simulink model "PowerSystem_FinalProject"  (R2020b)
settings: Solver=ode8  StartTime=0.0  StopTime=10  RelTol=1e-4  EnableMultiTasking=on
PreLoadFcn:
  | ct = 1.083
undefined symbols (not defined in the file): D1, Delta
libraries: powerlib x43, powerlib_meascontrol x9, sps_avr x3
settings Model: Creator=jp536285  LastModifiedBy=Arda
settings DataIOCC: SaveFormat=Array  SaveOutput=off  SaveTime=off  ReturnWorkspaceOutputs=off
settings OptimizationCC: LifeSpan=inf
settings DebuggingCC: UnderspecifiedInitializationDetection=Classic  MergeDetectMultiDrivingBlocksExec=none  SolverPrmCheckMsg=warning  UnconnectedInputMsg=none  UnconnectedOutputMsg=none  UnconnectedLineMsg=none  StateNameClashWarn=warning  SFUnexpectedBacktrackingDiag=warning  SFNoUnconditionalDefaultTransitionDiag=warning  SFExecutionAtInitializationDiag=none  ArithmeticOperatorsInVariantConditions=warning
settings HardwareCC: ProdBitPerPointer=32  ProdBitPerSizeT=32  ProdBitPerPtrDiffT=32  ProdLargestAtomicFloat=None  ProdIntDivRoundTo=Undefined  ProdEndianess=Unspecified  ProdWordSize=32  ProdHWDeviceType=32-bit Generic
settings ModelReferenceCC: PropagateSignalLabelsOutOfModel=off
settings SFSimCC: SimUseLocalCustomCode=off  CustomCodeUndefinedFunction=UseInterfaceOnly
settings RTWCC: RTWUseLocalCustomCode=off
settings CodeAppCC: StateflowObjectComments=on
settings GRTTargetCC: TargetLangStandard=C89/C90 (ANSI)
settings ConfigComp: CovMetricSettings=dw  CovSaveCumulativeToWorkspaceVar=on  CovSaveSingleToWorkspaceVar=on  CovExternalEMLEnable=off
settings SimscapeCC: SimscapeNormalizeSystem=off

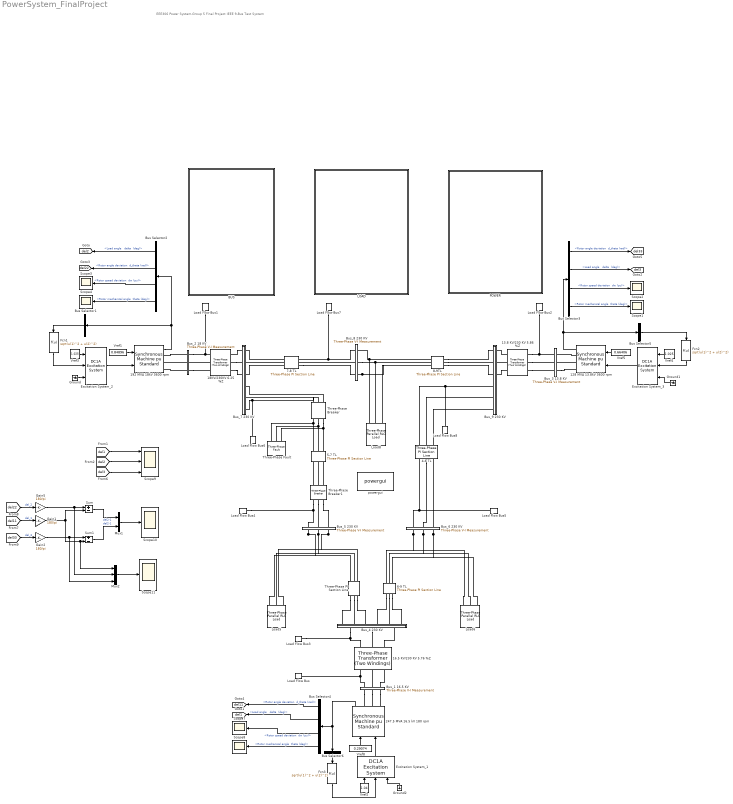
== system PowerSystem_FinalProject ==
  note: EEE306 Power System-Group 5
      |                      Final Project
      |             IEEE 9-Bus Test System
  128 MVA 13.8kV 3600 rpm : powerlib/Machines/Synchronous Machine pu Standard  PresetModel=No  MechanicalLoad=Mechanical power Pm  ShowDetailedParameters=on  RotorType=Round  Units=per unit standard parameters  MeasurementBus=off  NominalParameters="[ 128e6  13.8e3   60 ]"  Reactances1=[ 1.68, 0.23206, 0.19, 1.61, 0.23206, 0.19, 0.314]  Reactances2="[ 1.305, 0.296, 0.252, 0.474,  0.243,  0.18 ]"  dAxisTimeConstants=Open-circuit  qAxisTimeConstants=Open-circuit  TimeConstants1="[ 4.4849  0.0681  0.1  ]"  TimeConstants2=[ 5.89, 0.001,0.6, 0.001 ]  TimeConstants3="[  4.49  0.0681  0.0513  ]"  TimeConstants4=[ 8.0, 0.03, 0.3371, 0.0295 ]  TimeConstants5=[ 1.01, 0.053, 0.1 ]  TimeConstants6=[ 1.3201, 0.023, 1.0, 0.07 ]  TimeConstants7="[  1.01  0.053  0.051266  ]"  TimeConstants8=[ 1.3201, 0.0231, 0.3371, 0.0295 ]  StatorResistance=1e-7  Mechanical="[ 2.35  0 1 ]"  PolePairs=1  InitialConditions=[0 -40.1892 0.648353 0.648353 0.648353 5.37848 -114.622 125.378 1.46611]  SetSaturation=off  Saturation=[0.6404,0.7127,0.8441,0.9214,0.9956,1.082,1.19,1.316,1.457;0.7,0.7698,0.8872,0.9466,0.9969,1.046,1.1,1.151,1.201]  LoadFlowParameters=[1 85000000 0 0 0]  TsPowergui=0  TsBlock=-1  IterativeModel=Trapezoidal non iterative  IterativeDiscreteModel=Trapezoidal non iterative  BusType=PV  Pref=85000000  Qref=0  Qmin=-Inf  Qmax=Inf  PLF=0  QLF=0
  13.8 KV/230 KV 5.86 %Z : powerlib/Elements/Three-Phase Transformer (Two Windings)  Winding1Connection=Delta (D1)  Winding2Connection=Yg  CoreType=Three single-phase transformers  SetSaturation=off  Hysteresis=off  DataFile='hysteresis'  SetInitialFlux=off  Measurements=None  UNITS=pu  NominalPower=[ 128e6 , 60 ]  Winding1=[ 13.8e3 , 1e-6 , 0 ]  Winding2=[ 230e3 , 1e-6, 0.0586 ]  Rm=500  Lm=500  L0=0.5  Saturation=[ 0,0 ; 0.0024,1.2 ; 1.0,1.52 ]  InitialFluxes=[ 0.8 , -0.8 , 0.7 ]  BreakLoop=off  DiscreteSolver=Trapezoidal iterative  DataType=off  TransfoNumber=1
  "16.5 KV/230 KV 5.76 %Z     " : powerlib/Elements/Three-Phase Transformer (Two Windings)  Winding1Connection=Delta (D1)  Winding2Connection=Yg  CoreType=Three single-phase transformers  SetSaturation=off  Hysteresis=off  DataFile='hysteresis'  SetInitialFlux=off  Measurements=None  UNITS=pu  NominalPower=[ 247.5e6 , 60 ]  Winding1=[ 16.5e3 , 1e-6, 0 ]  Winding2=[ 230e3 ,1e-6, 0.0576 ]  Rm=500  Lm=500  L0=0.5  Saturation=[ 0,0 ; 0.0024,1.2 ; 1.0,1.52 ]  InitialFluxes=[ 0.8 , -0.8 , 0.7 ]  BreakLoop=off  DiscreteSolver=Trapezoidal iterative  DataType=off  TransfoNumber=1
  18KV/230KV 6.25 %Z : powerlib/Elements/Three-Phase Transformer (Two Windings)  Winding1Connection=Delta (D1)  Winding2Connection=Yg  CoreType=Three single-phase transformers  SetSaturation=off  Hysteresis=off  DataFile='hysteresis'  SetInitialFlux=off  Measurements=None  UNITS=pu  NominalPower=[ 192e6, 60 ]  Winding1=[ 18e3 , 1e-6 , 0]  Winding2=[ 230e3 , 1e-6, 0.0625 ]  Rm=500  Lm=500  L0=0.5  Saturation=[ 0,0 ; 0.0024,1.2 ; 1.0,1.52 ]  InitialFluxes=[ 0.8 , -0.8 , 0.7 ]  BreakLoop=off  DiscreteSolver=Trapezoidal iterative  DataType=off  TransfoNumber=1
  192 MVA 18kV 3600 rpm : powerlib/Machines/Synchronous Machine pu Standard  PresetModel=No  MechanicalLoad=Mechanical power Pm  ShowDetailedParameters=on  RotorType=Round  Units=per unit standard parameters  MeasurementBus=off  NominalParameters="[ 192e6  18e3   60 ]"  Reactances1=[ 1.72, 0.23, 0.1728,1.65, 0.23, 0.1728, 0.4224 ]  Reactances2="[ 1.305, 0.296, 0.252, 0.474,  0.243,  0.18 ]"  dAxisTimeConstants=Open-circuit  qAxisTimeConstants=Open-circuit  TimeConstants1="[ 4.4849  0.0681  0.1  ]"  TimeConstants2=[ 6, 0.001, 0.53, 0.001]  TimeConstants3="[  4.49  0.0681  0.0513  ]"  TimeConstants4=[ 8.0, 0.03, 0.3371, 0.0295 ]  TimeConstants5=[ 1.01, 0.053, 0.1 ]  TimeConstants6=[ 1.3201, 0.023, 1.0, 0.07 ]  TimeConstants7="[  1.01  0.053  0.051266  ]"  TimeConstants8=[ 1.3201, 0.0231, 0.3371, 0.0295 ]  StatorResistance=1e-7  Mechanical="[ 3.33  0 1 ]"  PolePairs=1  InitialConditions=[0 -30.0005 0.828257 0.828257 0.828257 6.94163 -113.058 126.942 1.7518]  SetSaturation=off  Saturation=[0.6404,0.7127,0.8441,0.9214,0.9956,1.082,1.19,1.316,1.457;0.7,0.7698,0.8872,0.9466,0.9969,1.046,1.1,1.151,1.201]  LoadFlowParameters=[1 163000000 0 0 0]  TsPowergui=0  TsBlock=-1  IterativeModel=Trapezoidal non iterative  IterativeDiscreteModel=Trapezoidal non iterative  BusType=PV  Pref=163000000  Qref=0  Qmin=-Inf  Qmax=Inf  PLF=0  QLF=0
  247.5 MVA 16.5 kV 180 rpm : powerlib/Machines/Synchronous Machine pu Standard  PresetModel=No  MechanicalLoad=Mechanical power Pm  ShowDetailedParameters=on  RotorType=Salient-pole  Units=per unit standard parameters  MeasurementBus=off  NominalParameters="[ 247.5e6  16500   60 ]"  Reactances1=[ 31 32 33 34 35 36 37 ]  Reactances2=[ 0.361, 0.1504, 0.099, 0.2398, 0.099, 0.062 ]  dAxisTimeConstants=Open-circuit  qAxisTimeConstants=Open-circuit  TimeConstants1=[8.96 0.001 0.001]  TimeConstants2=[]  TimeConstants3=[]  TimeConstants4=[]  TimeConstants5=[ 1.01, 0.053, 0.31 ]  TimeConstants6=[]  TimeConstants7=[]  TimeConstants8=[]  StatorResistance=1e-7  Mechanical=[9.55 0 20]  PolePairs=20  InitialConditions=[0 -86.3582 0.284957 0.284957 0.284957 -11.1761 -131.176 108.824 1.06421]  SetSaturation=off  Saturation=[0.6404,0.7127,0.8441,0.9214,0.9956,1.082,1.19,1.316,1.457;0.7,0.7698,0.8872,0.9466,0.9969,1.046,1.1,1.151,1.201]  LoadFlowParameters=[2 71000000 0 0]  TsPowergui=0  TsBlock=-1  IterativeModel=Trapezoidal non iterative  IterativeDiscreteModel=Trapezoidal non iterative  BusType=swing  Pref=150000000  Qref=0  Qmin=-Inf  Qmax=Inf  PLF=0  QLF=0
      settings: AttributesFormatString=\n\n
  4-6 TL : powerlib/Elements/Three-Phase PI Section Line  LConnTagsString=a|b|c  RConnTagsString=A|B|C  Length=97.336  Frequency=60  Resistances=[9.24e-2 9.24e-1]  Inductances=[1.40e-3 3.98e-3]  Capacitances=[8.14e-9 4.88e-9]
  5-7 TL : powerlib/Elements/Three-Phase PI Section Line  LConnTagsString=a|b|c  RConnTagsString=A|B|C  Length=170.338  Frequency=60  Resistances=[9.94e-2 9.94e-1]  Inductances=[1.4e-3 3.98e-3]  Capacitances=[9.01e-9 5.41e-9]
  6-9 TL : powerlib/Elements/Three-Phase PI Section Line  LConnTagsString=a|b|c  RConnTagsString=A|B|C  Length=179.86  Frequency=60  Resistances=[1.15e-1 1.15]  Inductances=[1.4e-3 3.98e-3]  Capacitances=[9.98e-9 5.99e-9]
  7-8 TL : powerlib/Elements/Three-Phase PI Section Line  LConnTagsString=a|b|c  RConnTagsString=A|B|C  Length=76.176  Frequency=60  Resistances=[5.90e-2 5.90e-1]  Inductances=[1.4e-3 3.98e-3]  Capacitances=[9.81e-9 5.89e-9]
  8-9TL : powerlib/Elements/Three-Phase PI Section Line  LConnTagsString=a|b|c  RConnTagsString=A|B|C  Length=106.646  Frequency=60  Resistances=[5.9e-2 5.9e-1]  Inductances=[1.4e-3 3.98e-3]  Capacitances=[9.83e-9 5.9e-9]
  "BUS " : Subsystem
  Bus Selector1 : BusSelector  OutputSignals="dq0 components.Stator voltage  vq (pu),dq0 components.Stator voltage  vd (pu)"  OutputAsBus=on
  Bus Selector2 : BusSelector  OutputSignals="Load angle   delta  (deg),Mechanical.Rotor angle deviation  d_theta (rad),Mechanical.Rotor speed deviation  dw (pu),Mechanical.Rotor mechanical angle  theta (deg)"
  Bus Selector3 : BusSelector  OutputSignals="Mechanical.Rotor angle deviation  d_theta (rad),Load angle   delta  (deg),Mechanical.Rotor speed deviation  dw (pu),Mechanical.Rotor mechanical angle  theta (deg)"
  Bus Selector4 : BusSelector  OutputSignals="Mechanical.Rotor angle deviation  d_theta (rad),Load angle   delta  (deg),Mechanical.Rotor speed deviation  dw (pu),Mechanical.Rotor mechanical angle  theta (deg)"
  Bus Selector5 : BusSelector  OutputSignals="dq0 components.Stator voltage  vq (pu),dq0 components.Stator voltage  vd (pu)"  OutputAsBus=on
  Bus Selector6 : BusSelector  OutputSignals="dq0 components.Stator voltage  vq (pu),dq0 components.Stator voltage  vd (pu)"  OutputAsBus=on
  Bus_1 16.5 KV : powerlib/Measurements/Three-Phase V-I Measurement  VoltageMeasurement=phase-to-phase  SetLabelV=on  LabelV=Vabc_1  Vpu=on  VpuLL=off  CurrentMeasurement=yes  SetLabelI=on  LabelI=Iabc_1  Ipu=on  Pbase=100e6  Vbase=16.5e3  OutputType=Complex  PhasorSimulation=off  PSBequivalent=0
  Bus_2 18 KV : powerlib/Measurements/Three-Phase V-I Measurement  VoltageMeasurement=phase-to-phase  SetLabelV=on  LabelV=Vabc_2  Vpu=on  VpuLL=off  CurrentMeasurement=yes  SetLabelI=on  LabelI=Iabc_2  Ipu=on  Pbase=100e6  Vbase=18e3  OutputType=Complex  PhasorSimulation=off  PSBequivalent=0
  Bus_3 13.8 KV : powerlib/Measurements/Three-Phase V-I Measurement  VoltageMeasurement=phase-to-phase  SetLabelV=on  LabelV=Vabc_3  Vpu=on  VpuLL=off  CurrentMeasurement=yes  SetLabelI=on  LabelI=Iabc_3  Ipu=on  Pbase=100e6  Vbase=13.8e3  OutputType=Complex  PhasorSimulation=off  PSBequivalent=0
  Bus_4 230 KV : Subsystem
  Bus_5 230 KV : powerlib/Measurements/Three-Phase V-I Measurement  VoltageMeasurement=phase-to-ground  SetLabelV=on  LabelV=Vabc_5  Vpu=on  VpuLL=off  CurrentMeasurement=yes  SetLabelI=on  LabelI=Iabc_5  Ipu=on  Pbase=100e6  Vbase=230e3  OutputType=Complex  PhasorSimulation=off  PSBequivalent=0
  Bus_6 230 KV : powerlib/Measurements/Three-Phase V-I Measurement  VoltageMeasurement=phase-to-ground  SetLabelV=on  LabelV=Vabc_6  Vpu=on  VpuLL=off  CurrentMeasurement=yes  SetLabelI=on  LabelI=Iabc_6  Ipu=on  Pbase=100e6  Vbase=230e3  OutputType=Complex  PhasorSimulation=off  PSBequivalent=0
  Bus_7 230 KV : Subsystem
  Bus_8 230 KV : powerlib/Measurements/Three-Phase V-I Measurement  VoltageMeasurement=phase-to-ground  SetLabelV=on  LabelV=Vabc_8  Vpu=on  VpuLL=off  CurrentMeasurement=yes  SetLabelI=on  LabelI=Iabc_8  Ipu=on  Pbase=100e6  Vbase=230e3  OutputType=Complex  PhasorSimulation=off  PSBequivalent=0
  Bus_9 230 KV : Subsystem
  Excitation System_2 : sps_avr/DC1A Excitation System  Tr=20e-3  KaTa=[20 0.2]  VRminmax=[ -4 4]  KfTf=[0.063 0.35]  TbTc=[0 0]  KeTe=[1 0.314]  Efd12=[3.1 2.3]  SeEfd12=[0.483 0.1394]  v0=[1.025 1.7518]  TsBlock=0
      settings: SourceProductBaseCode=PS
  Excitation System_1 : sps_avr/DC1A Excitation System  Tr=20e-3  KaTa=[20 0.2]  VRminmax=[ -3 3]  KfTf=[0.063 0.35]  TbTc=[0 0]  KeTe=[1 0.314]  Efd12=[3.1 2.3]  SeEfd12=[0.483 0.1394]  v0=[1.04 1.0642]  TsBlock=0
      settings: SourceProductBaseCode=PS
  Excitation System_3 : sps_avr/DC1A Excitation System  Tr=20e-3  KaTa=[20 0.2]  VRminmax=[-4 4]  KfTf=[0.063 0.35]  TbTc=[0 0]  KeTe=[1 0.314]  Efd12=[3.1 2.3]  SeEfd12=[0.483 0.1394]  v0=[1.025 1.4661]  TsBlock=0
      settings: SourceProductBaseCode=PS
  Fcn1 : Fcn  Expr=sqrt(u(1)^2 + u(2)^2)
  Fcn2 : Fcn  Expr=sqrt(u(1)^2 + u(2)^2)
  Fcn3 : Fcn  Expr=sqrt(u(1)^2 + u(2)^2)
  Gain1 : Gain  Gain=180/pi
  Gain2 : Gain  Gain=180/pi
  Gain5 : Gain  Gain=180/pi
  Ground : Ground
  Ground1 : Ground
  Ground2 : Ground
  LOAD : Subsystem
  Load Flow Bus : powerlib/Measurements/Load Flow Bus  LConnTagsString=a  Phases=single  Connectors=on one side  ID=BUS_1  Vbase=16.5e3  Vref=1.04  Vangle=0  VLF=1.04  VLFb=1  VLFc=1  angleLF=0  angleLFb=0  angleLFc=0
      settings: AttributesFormatString=%<ID>\n%<Vbase>V\n%<VLF>pu\n%<angleLF>deg.
  Load Flow Bus1 : powerlib/Measurements/Load Flow Bus  LConnTagsString=a  Phases=single  Connectors=on one side  ID=BUS_2  Vbase=18e3  Vref=1.025  Vangle=0  VLF=1.025  VLFb=1  VLFc=1  angleLF=6.743  angleLFb=0  angleLFc=0
      settings: AttributesFormatString=%<ID>\n%<Vbase>V\n%<VLF>pu\n%<angleLF>deg.
  Load Flow Bus2 : powerlib/Measurements/Load Flow Bus  LConnTagsString=a  Phases=single  Connectors=on one side  ID=BUS_3  Vbase=13.8e3  Vref=1.025  Vangle=0  VLF=1.025  VLFb=1  VLFc=1  angleLF=3.158  angleLFb=0  angleLFc=0
      settings: AttributesFormatString=%<ID>\n%<Vbase>V\n%<VLF>pu\n%<angleLF>deg.
  Load Flow Bus3 : powerlib/Measurements/Load Flow Bus  LConnTagsString=a  Phases=single  Connectors=on one side  ID=BUS_4  Vbase=230e3  Vref=1  Vangle=0  VLF=1.037  VLFb=1  VLFc=1  angleLF=29.12  angleLFb=0  angleLFc=0
      settings: AttributesFormatString=%<ID>\n%<Vbase>V\n%<VLF>pu\n%<angleLF>deg.
  Load Flow Bus4 : powerlib/Measurements/Load Flow Bus  LConnTagsString=a  Phases=single  Connectors=on one side  ID=BUS_5  Vbase=230e3  Vref=1  Vangle=0  VLF=1.004  VLFb=1  VLFc=1  angleLF=26.79  angleLFb=0  angleLFc=0
      settings: AttributesFormatString=%<ID>\n%<Vbase>V\n%<VLF>pu\n%<angleLF>deg.
  Load Flow Bus5 : powerlib/Measurements/Load Flow Bus  LConnTagsString=a  Phases=single  Connectors=on one side  ID=BUS_6  Vbase=230e3  Vref=1  Vangle=0  VLF=1.017  VLFb=1  VLFc=1  angleLF=27.3  angleLFb=0  angleLFc=0
      settings: AttributesFormatString=%<ID>\n%<Vbase>V\n%<VLF>pu\n%<angleLF>deg.
  Load Flow Bus6 : powerlib/Measurements/Load Flow Bus  LConnTagsString=a  Phases=single  Connectors=on one side  ID=BUS_7  Vbase=230e3  Vref=1  Vangle=0  VLF=1.027  VLFb=1  VLFc=1  angleLF=33.86  angleLFb=0  angleLFc=0
      settings: AttributesFormatString=%<ID>\n%<Vbase>V\n%<VLF>pu\n%<angleLF>deg.
  Load Flow Bus7 : powerlib/Measurements/Load Flow Bus  LConnTagsString=a  Phases=single  Connectors=on one side  ID=BUS_8  Vbase=230e3  Vref=1  Vangle=0  VLF=1.014  VLFb=1  VLFc=1  angleLF=30.3  angleLFb=0  angleLFc=0
      settings: AttributesFormatString=%<ID>\n%<Vbase>V\n%<VLF>pu\n%<angleLF>deg.
  Load Flow Bus8 : powerlib/Measurements/Load Flow Bus  LConnTagsString=a  Phases=single  Connectors=on one side  ID=BUS_9  Vbase=230e3  Vref=1  Vangle=0  VLF=1.027  VLFb=1  VLFc=1  angleLF=31.05  angleLFb=0  angleLFc=0
      settings: AttributesFormatString=%<ID>\n%<Vbase>V\n%<VLF>pu\n%<angleLF>deg.
  Load5 : powerlib/Elements/Three-Phase Parallel RLC Load  LConnTagsString=A|B|C  Configuration=Y (grounded)  NominalVoltage=(230000)*1.00389  Vabc=[1e3 1e3 1e3]  Vabcp=[1e3 1e3 1e3]  NominalFrequency=60  UnbalancedPower=off  ActivePower=125e6  InductivePower=50e6  CapacitivePower=0  Pabc=[10e3 9e3 11e3]  QLabc=[100 90 110]  QCabc=[100 90 110]  Pabcp=[10e3 9e3 11e3]  QLabcp=[100 90 110]  QCabcp=[100 90 110]  Measurements=Branch voltages and currents  LoadType=constant PQ
  Load6 : powerlib/Elements/Three-Phase Parallel RLC Load  LConnTagsString=A|B|C  Configuration=Y (grounded)  NominalVoltage=(230000)*1.01696  Vabc=[1e3 1e3 1e3]  Vabcp=[1e3 1e3 1e3]  NominalFrequency=60  UnbalancedPower=off  ActivePower=90e6  InductivePower=30e6  CapacitivePower=0  Pabc=[10e3 9e3 11e3]  QLabc=[100 90 110]  QCabc=[100 90 110]  Pabcp=[10e3 9e3 11e3]  QLabcp=[100 90 110]  QCabcp=[100 90 110]  Measurements=Branch voltages and currents  LoadType=constant PQ
  Load8 : powerlib/Elements/Three-Phase Parallel RLC Load  LConnTagsString=A|B|C  Configuration=Y (grounded)  NominalVoltage=(230000)*1.0136  Vabc=[1e3 1e3 1e3]  Vabcp=[1e3 1e3 1e3]  NominalFrequency=60  UnbalancedPower=off  ActivePower=100e6  InductivePower=35e6  CapacitivePower=0  Pabc=[10e3 9e3 11e3]  QLabc=[100 90 110]  QCabc=[100 90 110]  Pabcp=[10e3 9e3 11e3]  QLabcp=[100 90 110]  QCabcp=[100 90 110]  Measurements=Branch voltages and currents  LoadType=constant PQ
  Mux1 : Mux  Inputs=2
  Mux2 : Mux  Inputs=3
  POWER : Subsystem
  Scope{1..4,7..8,10..11} (8 alike) : Scope
  Scope9 : Scope  NumInputPorts=3
  Sum : Sum  Inputs=+-
  Sum1 : Sum  Inputs=+-
  Three-Phase PI Section Line : powerlib/Elements/Three-Phase PI Section Line  LConnTagsString=a|b|c  RConnTagsString=A|B|C  Length=89.93  Frequency=60  Resistances=[5.88e-2 5.88e-1]  Inductances=[1.4e-3 3.98e-3]  Capacitances=[9.81e-9 5.89e-9]
  Three-Phase Breaker : powerlib/Elements/Three-Phase Breaker  InitialState=closed  SwitchA=on  SwitchB=on  SwitchC=on  SwitchTimes=[ct]  External=off  BreakerResistance=0.001  SnubberResistance=1e7  SnubberCapacitance=inf  Measurements=None
  Three-Phase Breaker1 : powerlib/Elements/Three-Phase Breaker  InitialState=closed  SwitchA=on  SwitchB=on  SwitchC=on  SwitchTimes=[ct]  External=off  BreakerResistance=0.001  SnubberResistance=1e7  SnubberCapacitance=inf  Measurements=None
  Three-Phase Fault : powerlib/Elements/Three-Phase Fault  InitialStates=0  FaultA=on  FaultB=on  FaultC=on  GroundFault=on  SwitchTimes=[1 ct]  External=off  SwitchStatus=NaN  FaultResistance=0.001  GroundResistance=0.01  SnubberResistance=1e6  SnubberCapacitance=inf  Measurements=None
  Vref1 : Constant  Value=0.84896
  Vref2 : Constant  Value=1.04
  Vref3 : Constant  Value=1.025
  Vref4 : Constant  Value=1.025
  Vref5 : Constant  Value=0.66406
  Vref8 : Constant  Value=0.29074
  powergui : powerlib/powergui  Priority=1  SimulationMode=Discrete  SampleTime=5e-5  frequency=60  Iterations=50  frequencyindice=60  Pbase=10e7  ErrMax=1e-05  UnitsV=kV  UnitsW=MW  buscounter=0  FunctionMessages=off  echomessages=off  EnableUseOfTLC=off  CurrentSourceSwitches=off  DisableSnubberDevices=off  DisableRonSwitches=off  DisableVfSwitches=off  DisplayEquations=off  AutomaticDiscreteSolvers=off  SolverType=Backward Euler  Interpol=off  ExternalGateDelay=off  methode=off  Ts=0  x0status=blocks  SPID=off  SwTol=0  HookPort=off  NonlinearTolerance=1e-4  nMaxIteration=100  ContinueOnMaxIteration=off  RestoreLinks=warning  ResistiveCurrentMeasurement=off  Frange=[0:2:500]  Ylog=off  Xlog=on  ShowGrid=off  save=off  variable=ZData  structure=0  ZoomFFT=off  StartTime=0.0  cycles=1  DisplayStyle=1  fundamental=60  FreqAxis=off  MaxFrequency=1000  frequencyindicesteady=1  RmsSteady=1  display=off
  tag scope: del11=global, del1=global, del22=global, del2=global, del33=global, del3=global
  wires:
  Vref5/1 -> 128 MVA 13.8kV 3600 rpm/1
  Excitation System_3/1 -> 128 MVA 13.8kV 3600 rpm/2
  192 MVA 18kV 3600 rpm/1 -> Bus Selector1/1, Bus Selector2/1
  Bus Selector2/1 -> [del2]  "<Load angle   delta  (deg)>"
  Bus Selector3/2 -> [del3]  "<Load angle   delta  (deg)>"
  128 MVA 13.8kV 3600 rpm/1 -> Bus Selector3/1, Bus Selector5/1
  247.5 MVA 16.5 kV 180 rpm/1 -> Bus Selector4/1, Bus Selector6/1
  Vref8/1 -> 247.5 MVA 16.5 kV 180 rpm/1
  Excitation System_1/1 -> 247.5 MVA 16.5 kV 180 rpm/2
  Bus Selector4/2 -> [del1]  "<Load angle   delta  (deg)>"
  Vref3/1 -> Excitation System_2/1
  Ground/1 -> Excitation System_2/3
  Vref4/1 -> Excitation System_3/1
  Ground1/1 -> Excitation System_3/3
  Vref2/1 -> Excitation System_1/1
  Bus Selector2/2 -> [del22]  "<Rotor angle deviation  d_theta (rad)>"
  Bus Selector4/1 -> [del11]  "<Rotor angle deviation  d_theta (rad)>"
  Bus Selector3/1 -> [del33]  "<Rotor angle deviation  d_theta (rad)>"
  Bus Selector2/3 -> Scope3/1  "<Rotor speed deviation  dw (pu)>"
  Vref1/1 -> 192 MVA 18kV 3600 rpm/1
  Bus Selector2/4 -> Scope4/1  "<Rotor mechanical angle  theta (deg)>"
  Bus Selector3/3 -> Scope2/1  "<Rotor speed deviation  dw (pu)>"
  Bus Selector3/4 -> Scope1/1  "<Rotor mechanical angle  theta (deg)>"
  Bus Selector4/3 -> Scope7/1  "<Rotor speed deviation  dw (pu)>"
  Bus Selector4/4 -> Scope8/1  "<Rotor mechanical angle  theta (deg)>"
  Bus Selector1/1 -> Fcn1/1
  Fcn1/1 -> Excitation System_2/2
  Excitation System_2/1 -> 192 MVA 18kV 3600 rpm/2
  Bus Selector5/1 -> Fcn2/1
  Fcn2/1 -> Excitation System_3/2
  Ground2/1 -> Excitation System_1/3
  Bus Selector6/1 -> Fcn3/1
  Fcn3/1 -> Excitation System_1/2
  [del3] -> Scope9/3
  [del2] -> Scope9/2
  [del1] -> Scope9/1
  Sum/1 -> Mux1/1  "del2-1"
  Sum1/1 -> Mux1/2  "del2-1"
  Mux1/1 -> Scope10/1
  Mux2/1 -> Scope11/1
  [del33] -> Gain2/1  "del_3"
  [del11] -> Gain1/1  "del_1"
  [del22] -> Gain5/1  "del_2"
  Gain5/1 -> Sum/1, Mux2/2
  Gain1/1 -> Mux2/1, Sum1/2, Sum/2
  Gain2/1 -> Sum1/1, Mux2/3
  connections:
  Bus_2 18 KV/LConn2 -- 192 MVA 18kV 3600 rpm/RConn2
  18KV/230KV 6.25 %Z/LConn2 -- Bus_2 18 KV/RConn2
  18KV/230KV 6.25 %Z/RConn2 -- Bus_7 230 KV/LConn2
  Bus_2 18 KV/RConn1 -- Load Flow Bus1/LConn1 -- 18KV/230KV 6.25 %Z/LConn1
  Bus_2 18 KV/RConn3 -- 18KV/230KV 6.25 %Z/LConn3
  Bus_7 230 KV/LConn1 -- 18KV/230KV 6.25 %Z/RConn1
  18KV/230KV 6.25 %Z/RConn3 -- Bus_7 230 KV/LConn3
  13.8 KV/230 KV 5.86 %Z/LConn1 -- Bus_3 13.8 KV/LConn1 -- Load Flow Bus2/LConn1
  13.8 KV/230 KV 5.86 %Z/LConn2 -- Bus_3 13.8 KV/LConn2
  13.8 KV/230 KV 5.86 %Z/LConn3 -- Bus_3 13.8 KV/LConn3
  Bus_1 16.5 KV/RConn1 -- 247.5 MVA 16.5 kV 180 rpm/RConn1
  Bus_1 16.5 KV/RConn2 -- 247.5 MVA 16.5 kV 180 rpm/RConn2
  Bus_1 16.5 KV/RConn3 -- 247.5 MVA 16.5 kV 180 rpm/RConn3
  Bus_1 16.5 KV/LConn3 -- "16.5 KV/230 KV 5.76 %Z     "/LConn3
  Bus_1 16.5 KV/LConn2 -- "16.5 KV/230 KV 5.76 %Z     "/LConn2
  13.8 KV/230 KV 5.86 %Z/RConn1 -- Bus_9 230 KV/RConn1
  13.8 KV/230 KV 5.86 %Z/RConn2 -- Bus_9 230 KV/RConn2
  13.8 KV/230 KV 5.86 %Z/RConn3 -- Bus_9 230 KV/RConn3
  Bus_4 230 KV/LConn1 -- "16.5 KV/230 KV 5.76 %Z     "/RConn1 -- Load Flow Bus3/LConn1
  Bus_4 230 KV/LConn2 -- "16.5 KV/230 KV 5.76 %Z     "/RConn2
  Load8/LConn1 -- Bus_8 230 KV/LConn1 -- 8-9TL/LConn1
  Bus_8 230 KV/LConn2 -- Load8/LConn2 -- 8-9TL/LConn2
  Bus_8 230 KV/LConn3 -- Load8/LConn3 -- 8-9TL/LConn3
  "16.5 KV/230 KV 5.76 %Z     "/RConn3 -- Bus_4 230 KV/LConn3
  Bus_5 230 KV/RConn1 -- Load5/LConn1 -- Three-Phase PI Section Line/LConn1
  Bus_5 230 KV/RConn2 -- Load5/LConn2 -- Three-Phase PI Section Line/LConn2
  Bus_5 230 KV/RConn3 -- Load5/LConn3 -- Three-Phase PI Section Line/LConn3
  Bus_6 230 KV/RConn1 -- Load6/LConn1 -- 6-9 TL/LConn1
  Bus_6 230 KV/RConn2 -- 6-9 TL/LConn2 -- Load6/LConn2
  Bus_6 230 KV/RConn3 -- 6-9 TL/LConn3 -- Load6/LConn3
  7-8 TL/LConn1 -- Bus_7 230 KV/RConn1
  7-8 TL/LConn2 -- Bus_7 230 KV/RConn2
  7-8 TL/LConn3 -- Bus_7 230 KV/RConn3
  Bus_8 230 KV/RConn1 -- 7-8 TL/RConn1 -- Load Flow Bus7/LConn1
  Bus_8 230 KV/RConn2 -- 7-8 TL/RConn2
  7-8 TL/RConn3 -- Bus_8 230 KV/RConn3
  8-9TL/RConn2 -- Bus_9 230 KV/LConn2
  8-9TL/RConn1 -- Bus_9 230 KV/LConn1
  8-9TL/RConn3 -- Bus_9 230 KV/LConn3
  Bus_7 230 KV/RConn6 -- Three-Phase Breaker/LConn1 -- Load Flow Bus6/LConn1
  4-6 TL/LConn1 -- Load Flow Bus8/LConn1 -- Bus_9 230 KV/LConn4
  Bus_9 230 KV/LConn5 -- 4-6 TL/LConn2
  Bus_6 230 KV/LConn1 -- 4-6 TL/RConn1 -- Load Flow Bus5/LConn1
  4-6 TL/RConn2 -- Bus_6 230 KV/LConn2
  Bus_6 230 KV/LConn3 -- 4-6 TL/RConn3
  4-6 TL/LConn3 -- Bus_9 230 KV/LConn6
  Three-Phase PI Section Line/RConn2 -- Bus_4 230 KV/RConn2
  Three-Phase PI Section Line/RConn1 -- Bus_4 230 KV/RConn1
  Three-Phase PI Section Line/RConn3 -- Bus_4 230 KV/RConn3
  6-9 TL/RConn2 -- Bus_4 230 KV/RConn5
  6-9 TL/RConn1 -- Bus_4 230 KV/RConn4
  6-9 TL/RConn3 -- Bus_4 230 KV/RConn6
  128 MVA 13.8kV 3600 rpm/RConn1 -- Bus_3 13.8 KV/RConn1
  128 MVA 13.8kV 3600 rpm/RConn2 -- Bus_3 13.8 KV/RConn2
  Bus_3 13.8 KV/RConn3 -- 128 MVA 13.8kV 3600 rpm/RConn3
  Bus_2 18 KV/LConn3 -- 192 MVA 18kV 3600 rpm/RConn3
  Bus_2 18 KV/LConn1 -- 192 MVA 18kV 3600 rpm/RConn1
  Bus_1 16.5 KV/LConn1 -- Load Flow Bus/LConn1 -- "16.5 KV/230 KV 5.76 %Z     "/LConn1
  Three-Phase Breaker/RConn2 -- Three-Phase Fault/LConn2 -- 5-7 TL/LConn2
  Three-Phase Breaker/RConn1 -- Three-Phase Fault/LConn1 -- 5-7 TL/LConn1
  Three-Phase Breaker/RConn3 -- Three-Phase Fault/LConn3 -- 5-7 TL/LConn3
  Three-Phase Breaker/LConn2 -- Bus_7 230 KV/RConn5
  Three-Phase Breaker/LConn3 -- Bus_7 230 KV/RConn4
  Three-Phase Breaker1/LConn2 -- 5-7 TL/RConn2
  Three-Phase Breaker1/RConn2 -- Bus_5 230 KV/LConn2
  Three-Phase Breaker1/LConn1 -- 5-7 TL/RConn1
  Three-Phase Breaker1/LConn3 -- 5-7 TL/RConn3
  Three-Phase Breaker1/RConn3 -- Bus_5 230 KV/LConn3
  Load Flow Bus4/LConn1 -- Three-Phase Breaker1/RConn1 -- Bus_5 230 KV/LConn1

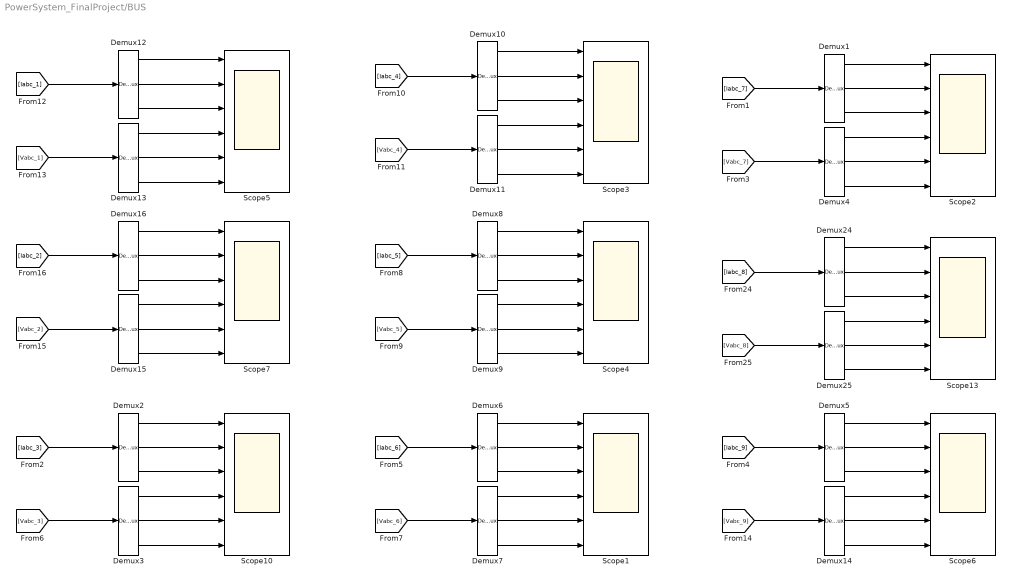
== system PowerSystem_FinalProject/BUS  ==
  Demux{1..16,24..25} (18 alike) : Demux  Outputs=3
  Scope{1..7,10,13} (9 alike) : Scope  NumInputPorts=6
  wires:
  Demux3/3 -> Scope10/6
  Demux2/3 -> Scope10/3
  Demux2/1 -> Scope10/1
  [Vabc_3] -> Demux3/1
  Demux2/2 -> Scope10/2
  Demux3/1 -> Scope10/4
  [Iabc_3] -> Demux2/1
  Demux3/2 -> Scope10/5
  Demux7/2 -> Scope1/5
  [Iabc_6] -> Demux6/1
  Demux7/1 -> Scope1/4
  Demux6/2 -> Scope1/2
  [Vabc_6] -> Demux7/1
  Demux6/1 -> Scope1/1
  Demux6/3 -> Scope1/3
  Demux7/3 -> Scope1/6
  Demux11/3 -> Scope3/6
  Demux10/3 -> Scope3/3
  Demux10/1 -> Scope3/1
  [Vabc_4] -> Demux11/1
  Demux10/2 -> Scope3/2
  Demux11/1 -> Scope3/4
  [Iabc_4] -> Demux10/1
  Demux11/2 -> Scope3/5
  Demux13/2 -> Scope5/5
  [Iabc_1] -> Demux12/1
  Demux13/1 -> Scope5/4
  Demux12/2 -> Scope5/2
  [Vabc_1] -> Demux13/1
  Demux12/1 -> Scope5/1
  Demux12/3 -> Scope5/3
  Demux13/3 -> Scope5/6
  Demux25/3 -> Scope13/6
  Demux24/3 -> Scope13/3
  Demux24/1 -> Scope13/1
  [Vabc_8] -> Demux25/1
  Demux24/2 -> Scope13/2
  Demux25/1 -> Scope13/4
  [Iabc_8] -> Demux24/1
  Demux25/2 -> Scope13/5
  Demux4/2 -> Scope2/5
  [Iabc_7] -> Demux1/1
  Demux4/1 -> Scope2/4
  Demux1/2 -> Scope2/2
  [Vabc_7] -> Demux4/1
  Demux1/1 -> Scope2/1
  Demux1/3 -> Scope2/3
  Demux4/3 -> Scope2/6
  Demux14/3 -> Scope6/6
  Demux5/3 -> Scope6/3
  Demux5/1 -> Scope6/1
  [Vabc_9] -> Demux14/1
  Demux5/2 -> Scope6/2
  Demux14/1 -> Scope6/4
  [Iabc_9] -> Demux5/1
  Demux14/2 -> Scope6/5
  Demux15/2 -> Scope7/5
  [Iabc_2] -> Demux16/1
  Demux15/1 -> Scope7/4
  Demux16/2 -> Scope7/2
  [Vabc_2] -> Demux15/1
  Demux16/1 -> Scope7/1
  Demux16/3 -> Scope7/3
  Demux15/3 -> Scope7/6
  Demux9/2 -> Scope4/5
  [Iabc_5] -> Demux8/1
  Demux9/1 -> Scope4/4
  Demux8/2 -> Scope4/2
  [Vabc_5] -> Demux9/1
  Demux8/1 -> Scope4/1
  Demux8/3 -> Scope4/3
  Demux9/3 -> Scope4/6

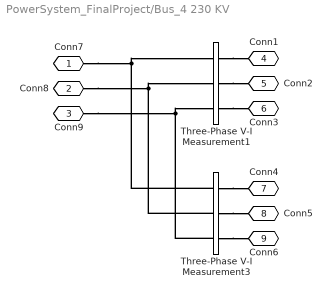
== system PowerSystem_FinalProject/Bus_4 230 KV ==
  Three-Phase V-I Measurement1 : powerlib/Measurements/Three-Phase V-I Measurement  VoltageMeasurement=phase-to-ground  SetLabelV=on  LabelV=Vabc_4  Vpu=on  VpuLL=off  CurrentMeasurement=yes  SetLabelI=on  LabelI=Iabc_4  Ipu=on  Pbase=100e6  Vbase=230e3  OutputType=Complex  PhasorSimulation=off  PSBequivalent=0
  Three-Phase V-I Measurement3 : powerlib/Measurements/Three-Phase V-I Measurement  VoltageMeasurement=phase-to-ground  SetLabelV=on  LabelV=Vabc_46  Vpu=on  VpuLL=off  CurrentMeasurement=yes  SetLabelI=on  LabelI=Iabc_46  Ipu=on  Pbase=100e6  Vbase=230e3  OutputType=Complex  PhasorSimulation=off  PSBequivalent=0
  Conn7 : PMIOPort  Side=Left
  Conn8 : PMIOPort  Port=2  Side=Left
  Conn9 : PMIOPort  Port=3  Side=Left
  Conn1 : PMIOPort  Port=4  Side=Right
  Conn2 : PMIOPort  Port=5  Side=Right
  Conn3 : PMIOPort  Port=6  Side=Right
  Conn4 : PMIOPort  Port=7  Side=Right
  Conn5 : PMIOPort  Port=8  Side=Right
  Conn6 : PMIOPort  Port=9  Side=Right
  connections:
  Three-Phase V-I Measurement3/LConn3 -- Conn9/RConn1 -- Three-Phase V-I Measurement1/LConn3
  Three-Phase V-I Measurement3/LConn2 -- Conn8/RConn1 -- Three-Phase V-I Measurement1/LConn2
  Three-Phase V-I Measurement3/LConn1 -- Conn7/RConn1 -- Three-Phase V-I Measurement1/LConn1
  Three-Phase V-I Measurement3/RConn3 -- Conn6/RConn1
  Three-Phase V-I Measurement1/RConn3 -- Conn3/RConn1
  Three-Phase V-I Measurement1/RConn1 -- Conn1/RConn1
  Three-Phase V-I Measurement1/RConn2 -- Conn2/RConn1
  Three-Phase V-I Measurement3/RConn1 -- Conn4/RConn1
  Three-Phase V-I Measurement3/RConn2 -- Conn5/RConn1

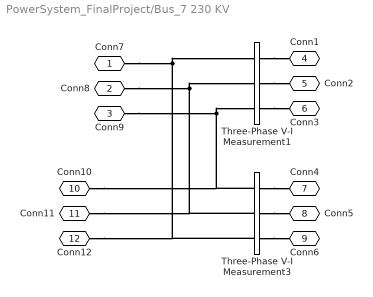
== system PowerSystem_FinalProject/Bus_7 230 KV ==
  Three-Phase V-I Measurement1 : powerlib/Measurements/Three-Phase V-I Measurement  VoltageMeasurement=phase-to-ground  SetLabelV=on  LabelV=Vabc_7  Vpu=on  VpuLL=off  CurrentMeasurement=yes  SetLabelI=on  LabelI=Iabc_7  Ipu=on  Pbase=100e6  Vbase=230e3  OutputType=Complex  PhasorSimulation=off  PSBequivalent=0
  Three-Phase V-I Measurement3 : powerlib/Measurements/Three-Phase V-I Measurement  VoltageMeasurement=phase-to-ground  SetLabelV=on  LabelV=Vab  Vpu=on  VpuLL=off  CurrentMeasurement=yes  SetLabelI=on  LabelI=Iab  Ipu=on  Pbase=100e6  Vbase=230e3  OutputType=Complex  PhasorSimulation=off  PSBequivalent=0
  Conn7 : PMIOPort  Side=Left
  Conn8 : PMIOPort  Port=2  Side=Left
  Conn9 : PMIOPort  Port=3  Side=Left
  Conn1 : PMIOPort  Port=4  Side=Right
  Conn2 : PMIOPort  Port=5  Side=Right
  Conn3 : PMIOPort  Port=6  Side=Right
  Conn4 : PMIOPort  Port=7  Side=Right
  Conn5 : PMIOPort  Port=8  Side=Right
  Conn6 : PMIOPort  Port=9  Side=Right
  Conn10 : PMIOPort  Port=10  Side=Left
  Conn11 : PMIOPort  Port=11  Side=Left
  Conn12 : PMIOPort  Port=12  Side=Left
  connections:
  Three-Phase V-I Measurement3/RConn2 -- Conn5/RConn1
  Three-Phase V-I Measurement3/RConn1 -- Conn4/RConn1
  Three-Phase V-I Measurement1/RConn2 -- Conn2/RConn1
  Three-Phase V-I Measurement1/RConn1 -- Conn1/RConn1
  Three-Phase V-I Measurement1/RConn3 -- Conn3/RConn1
  Three-Phase V-I Measurement3/RConn3 -- Conn6/RConn1
  Conn7/RConn1 -- Three-Phase V-I Measurement3/LConn3 -- Conn12/RConn1 -- Three-Phase V-I Measurement1/LConn1
  Conn8/RConn1 -- Three-Phase V-I Measurement3/LConn2 -- Conn11/RConn1 -- Three-Phase V-I Measurement1/LConn2
  Conn9/RConn1 -- Conn10/RConn1 -- Three-Phase V-I Measurement3/LConn1 -- Three-Phase V-I Measurement1/LConn3

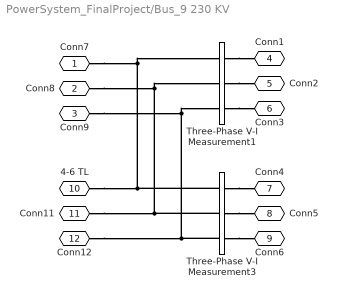
== system PowerSystem_FinalProject/Bus_9 230 KV ==
  Three-Phase V-I Measurement1 : powerlib/Measurements/Three-Phase V-I Measurement  VoltageMeasurement=phase-to-ground  SetLabelV=on  LabelV=Vabc_9  Vpu=on  VpuLL=off  CurrentMeasurement=yes  SetLabelI=on  LabelI=Iabc_9  Ipu=on  Pbase=100e6  Vbase=230e3  OutputType=Complex  PhasorSimulation=off  PSBequivalent=0
  Three-Phase V-I Measurement3 : powerlib/Measurements/Three-Phase V-I Measurement  VoltageMeasurement=phase-to-ground  SetLabelV=on  LabelV=Vabc  Vpu=on  VpuLL=off  CurrentMeasurement=yes  SetLabelI=on  LabelI=Iabc  Ipu=on  Pbase=100e6  Vbase=230e3  OutputType=Complex  PhasorSimulation=off  PSBequivalent=0
  Conn7 : PMIOPort  Side=Left
  Conn8 : PMIOPort  Port=2  Side=Left
  Conn9 : PMIOPort  Port=3  Side=Left
  Conn1 : PMIOPort  Port=4  Side=Right
  Conn2 : PMIOPort  Port=5  Side=Right
  Conn3 : PMIOPort  Port=6  Side=Right
  Conn4 : PMIOPort  Port=7  Side=Right
  Conn5 : PMIOPort  Port=8  Side=Right
  Conn6 : PMIOPort  Port=9  Side=Right
  4-6 TL : PMIOPort  Port=10  Side=Left
  Conn11 : PMIOPort  Port=11  Side=Left
  Conn12 : PMIOPort  Port=12  Side=Left
  connections:
  Conn12/RConn1 -- Three-Phase V-I Measurement3/LConn3 -- Conn9/RConn1 -- Three-Phase V-I Measurement1/LConn3
  Conn11/RConn1 -- Three-Phase V-I Measurement3/LConn2 -- Conn8/RConn1 -- Three-Phase V-I Measurement1/LConn2
  4-6 TL/RConn1 -- Three-Phase V-I Measurement3/LConn1 -- Conn7/RConn1 -- Three-Phase V-I Measurement1/LConn1
  Three-Phase V-I Measurement3/RConn3 -- Conn6/RConn1
  Three-Phase V-I Measurement1/RConn3 -- Conn3/RConn1
  Three-Phase V-I Measurement1/RConn1 -- Conn1/RConn1
  Three-Phase V-I Measurement1/RConn2 -- Conn2/RConn1
  Three-Phase V-I Measurement3/RConn1 -- Conn4/RConn1
  Three-Phase V-I Measurement3/RConn2 -- Conn5/RConn1

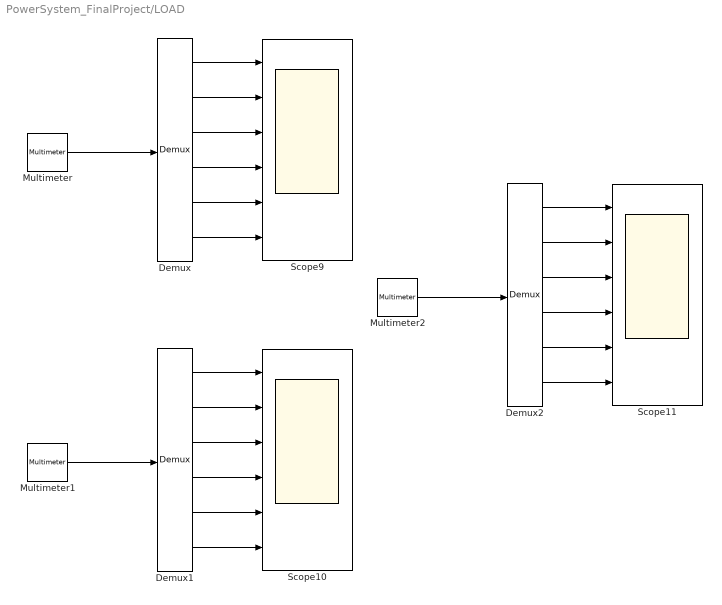
== system PowerSystem_FinalProject/LOAD ==
  Demux : Demux  Outputs=6
  Demux1 : Demux  Outputs=6
  Demux2 : Demux  Outputs=6
  Multimeter : powerlib/Measurements/Multimeter  PhasorSimulation=off  OutputType=Complex  sel=[1 2 3 10 11 12]  L=18  Gain=[1 1 1 1 1 1]  yselected={'Uag: Load5','Ubg: Load5','Ucg: Load5','Iag: Load5','Ibg: Load5','Icg: Load5'};  PSBOutputType=1  PSBequivalent=0  AxesSetting=[0,0.1,-100,100]  Display=0  SavedBlockNames=-11
  Multimeter1 : powerlib/Measurements/Multimeter  PhasorSimulation=off  OutputType=Complex  sel=[4 5 6 13 14 15]  L=18  Gain=[1 1 1 1 1 1]  yselected={'Uag: Load6','Ubg: Load6','Ucg: Load6','Iag: Load6','Ibg: Load6','Icg: Load6'};  PSBOutputType=1  PSBequivalent=0  AxesSetting=[0,0.1,-100,100]  Display=0  SavedBlockNames=-11
  Multimeter2 : powerlib/Measurements/Multimeter  PhasorSimulation=off  OutputType=Complex  sel=[7 8 9 16 17 18]  L=18  Gain=[1 1 1 1 1 1]  yselected={'Uag: Load8','Ubg: Load8','Ucg: Load8','Iag: Load8','Ibg: Load8','Icg: Load8'};  PSBOutputType=1  PSBequivalent=0  AxesSetting=[0,0.1,-100,100]  Display=0  SavedBlockNames=-11
  Scope10 : Scope  NumInputPorts=6
  Scope11 : Scope  NumInputPorts=6
  Scope9 : Scope  NumInputPorts=6
  wires:
  Demux/4 -> Scope9/4
  Demux/3 -> Scope9/3
  Demux2/5 -> Scope11/5
  Demux1/1 -> Scope10/1
  Multimeter/1 -> Demux/1
  Demux/5 -> Scope9/5
  Demux2/4 -> Scope11/4
  Demux2/1 -> Scope11/1
  Demux/1 -> Scope9/1
  Demux1/3 -> Scope10/3
  Demux/2 -> Scope9/2
  Demux1/6 -> Scope10/6
  Demux1/5 -> Scope10/5
  Demux1/4 -> Scope10/4
  Demux1/2 -> Scope10/2
  Multimeter1/1 -> Demux1/1
  Demux/6 -> Scope9/6
  Multimeter2/1 -> Demux2/1
  Demux2/2 -> Scope11/2
  Demux2/3 -> Scope11/3
  Demux2/6 -> Scope11/6

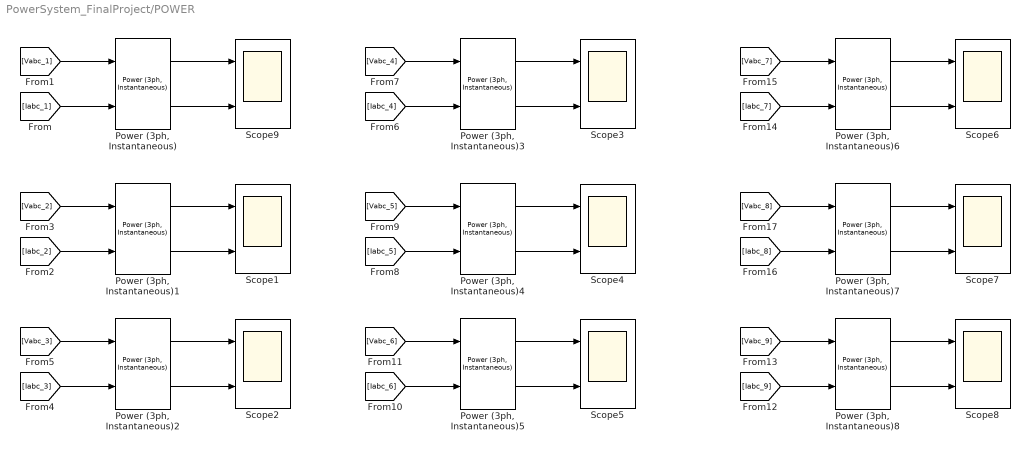
== system PowerSystem_FinalProject/POWER ==
  Power (3ph, Instantaneous){,1..8} (9 alike) : powerlib_meascontrol/Measurements/Power (3ph, Instantaneous)
  Scope{1..9} (9 alike) : Scope  NumInputPorts=2
  wires:
  "Power (3ph, Instantaneous)"/1 -> Scope9/1
  "Power (3ph, Instantaneous)"/2 -> Scope9/2
  [Iabc_1] -> "Power (3ph, Instantaneous)"/2
  [Vabc_1] -> "Power (3ph, Instantaneous)"/1
  [Vabc_2] -> "Power (3ph, Instantaneous)1"/1
  [Iabc_2] -> "Power (3ph, Instantaneous)1"/2
  "Power (3ph, Instantaneous)1"/2 -> Scope1/2
  "Power (3ph, Instantaneous)1"/1 -> Scope1/1
  "Power (3ph, Instantaneous)2"/1 -> Scope2/1
  "Power (3ph, Instantaneous)2"/2 -> Scope2/2
  [Iabc_3] -> "Power (3ph, Instantaneous)2"/2
  [Vabc_3] -> "Power (3ph, Instantaneous)2"/1
  [Vabc_4] -> "Power (3ph, Instantaneous)3"/1
  [Iabc_4] -> "Power (3ph, Instantaneous)3"/2
  "Power (3ph, Instantaneous)3"/2 -> Scope3/2
  "Power (3ph, Instantaneous)3"/1 -> Scope3/1
  "Power (3ph, Instantaneous)4"/1 -> Scope4/1
  "Power (3ph, Instantaneous)4"/2 -> Scope4/2
  [Iabc_5] -> "Power (3ph, Instantaneous)4"/2
  [Vabc_5] -> "Power (3ph, Instantaneous)4"/1
  [Vabc_6] -> "Power (3ph, Instantaneous)5"/1
  [Iabc_6] -> "Power (3ph, Instantaneous)5"/2
  "Power (3ph, Instantaneous)5"/2 -> Scope5/2
  "Power (3ph, Instantaneous)5"/1 -> Scope5/1
  "Power (3ph, Instantaneous)8"/1 -> Scope8/1
  "Power (3ph, Instantaneous)8"/2 -> Scope8/2
  [Iabc_9] -> "Power (3ph, Instantaneous)8"/2
  [Vabc_9] -> "Power (3ph, Instantaneous)8"/1
  [Vabc_8] -> "Power (3ph, Instantaneous)7"/1
  [Iabc_8] -> "Power (3ph, Instantaneous)7"/2
  "Power (3ph, Instantaneous)7"/2 -> Scope7/2
  "Power (3ph, Instantaneous)7"/1 -> Scope7/1
  "Power (3ph, Instantaneous)6"/1 -> Scope6/1
  "Power (3ph, Instantaneous)6"/2 -> Scope6/2
  [Iabc_7] -> "Power (3ph, Instantaneous)6"/2
  [Vabc_7] -> "Power (3ph, Instantaneous)6"/1
